simulink model "lab2"  (R2025b)
settings: Solver=VariableStepAuto  StartTime=0.0  StopTime=10.0  RelTol=1e-3
model workspace (MAT data in the model file):
  b = Simulink.Parameter
  b.Complexity = 'real'
  b.Dimensions = [0 0]
  b.DataType = 'auto'
undefined symbols (not defined in the file): Kd, Ki, Kp
settings Model: Creator=getrj  LastModifiedBy=owenm

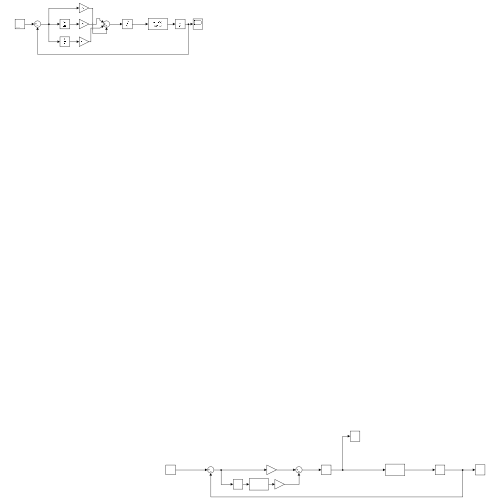
[thumbnail: Simulink's stored preview of the top-level diagram]
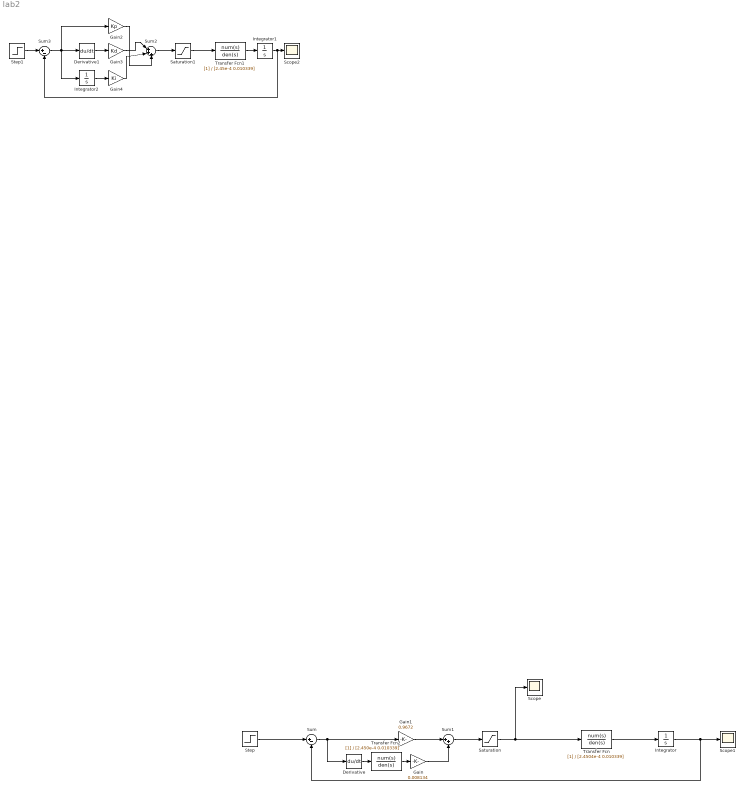
== system lab2 ==
  Derivative : Derivative
  Derivative1 : Derivative
  Gain : Gain  Gain=0.008134
  Gain1 : Gain  Gain=0.9672
  Gain2 : Gain  Gain=Kp
  Gain3 : Gain  Gain=Kd
  Gain4 : Gain  Gain=Ki
  Integrator : Integrator
  Integrator1 : Integrator
  Integrator2 : Integrator
  Saturation : Saturate  UpperLimit=10  LowerLimit=-10
  Saturation1 : Saturate  UpperLimit=10  LowerLimit=-10
  Scope : Scope
      settings: ActiveDisplayYMinimum=-1.0129203936463997  ActiveDisplayYMaximum=1.1872133770718221
  Scope1 : Scope
      settings: ActiveDisplayYMinimum=-0.0740190078435875  ActiveDisplayYMaximum=1.0869922838518802
  Scope2 : Scope
      settings: ActiveDisplayYMinimum=-27826.407492225706  ActiveDisplayYMaximum=38171.94016672868  DataLoggingVariableName=ScopeData2
  Step : Step  Time=0  SampleTime=0
  Step1 : Step  After=2  SampleTime=0
  Sum : Sum  Inputs=|+-
  Sum1 : Sum  Inputs=|++
  Sum2 : Sum  Inputs=|+++
  Sum3 : Sum  Inputs=|+-
  Transfer Fcn : TransferFcn  Denominator=[2.4504e-4 0.010339]
  Transfer Fcn1 : TransferFcn  Denominator=[2.45e-4 0.010339]
  Transfer Fcn2 : TransferFcn  Denominator=[2.450e-4 0.010339]
  wires:
  Step/1 -> Sum/1
  Sum/1 -> Derivative/1, Gain1/1
  Gain1/1 -> Sum1/1
  Gain/1 -> Sum1/2
  Sum1/1 -> Saturation/1
  Saturation/1 -> Transfer Fcn/1, Scope/1
  Transfer Fcn/1 -> Integrator/1
  Integrator/1 -> Sum/2, Scope1/1
  Derivative/1 -> Transfer Fcn2/1
  Transfer Fcn2/1 -> Gain/1
  Transfer Fcn1/1 -> Integrator1/1
  Saturation1/1 -> Transfer Fcn1/1
  Sum2/1 -> Saturation1/1
  Gain4/1 -> Sum2/2
  Gain3/1 -> Sum2/1
  Gain2/1 -> Sum2/3
  Integrator2/1 -> Gain4/1
  Derivative1/1 -> Gain3/1
  Sum3/1 -> Gain2/1, Integrator2/1, Derivative1/1
  Integrator1/1 -> Sum3/2, Scope2/1
  Step1/1 -> Sum3/1
